simulink model "eVTOL"  (R2025a)
settings: Solver=VariableStepAuto  StartTime=0.0  StopTime=10  RelTol=1e-3
values from neighbouring files (symbols this model uses):
  A = [0 1 0 0 0 0 ... (first row only)    [QRCalculation.m]    (also in QRCalculation2.m = sys.A)
  B = [0 0 0 ... (first row only)    [QRCalculation.m]    (also in QRCalculation2.m = sys.B)
  K = lqr(A,B,Q,R)    [QRCalculation.m]    (also in QRCalculation2.m)
  T = [1 0 0 0 0 0 ... (first row only)    [QRCalculation2.m]
  u0 = [w_trim_vec(1);w_trim_vec(2);w_trim_vec(3);w_trim_vec(4);        eta_trim;eta_trim;eta_trim;eta_trim;        gamma_trim;gamma_trim;gamma_trim;gamma_trim]    [QRCalculation2.m]
undefined symbols (not defined in the file or in its folder): magnitude, Rotor
libraries: aerolibconvert2 x6, shared6dof x1, sharedtransform x1
settings Model: Creator=Administrator  LastModifiedBy=zozo
settings SolverCC: AlgebraicLoopSolver=TrustRegion
settings DataIOCC: ReturnWorkspaceOutputs=off
settings DebuggingCC: UnconnectedInputMsg=warning  UnconnectedOutputMsg=warning  UnconnectedLineMsg=warning  ArithmeticOperatorsInVariantConditions=warning
settings ModelReferenceCC: EnableRefExpFcnMdlSchedulingChecks=on
settings SFSimCC: SimUseLocalCustomCode=off  CustomCodeUndefinedFunction=UseInterfaceOnly
settings RTWCC: RTWUseLocalCustomCode=off  GPUComputeCapability=3.5
settings CodeAppCC: StateflowObjectComments=on

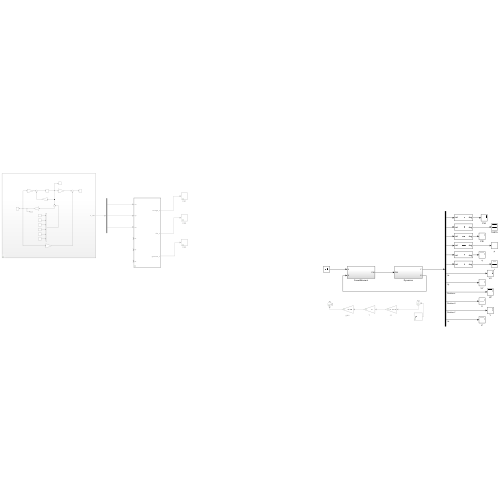
[thumbnail: Simulink's stored preview of the top-level diagram]
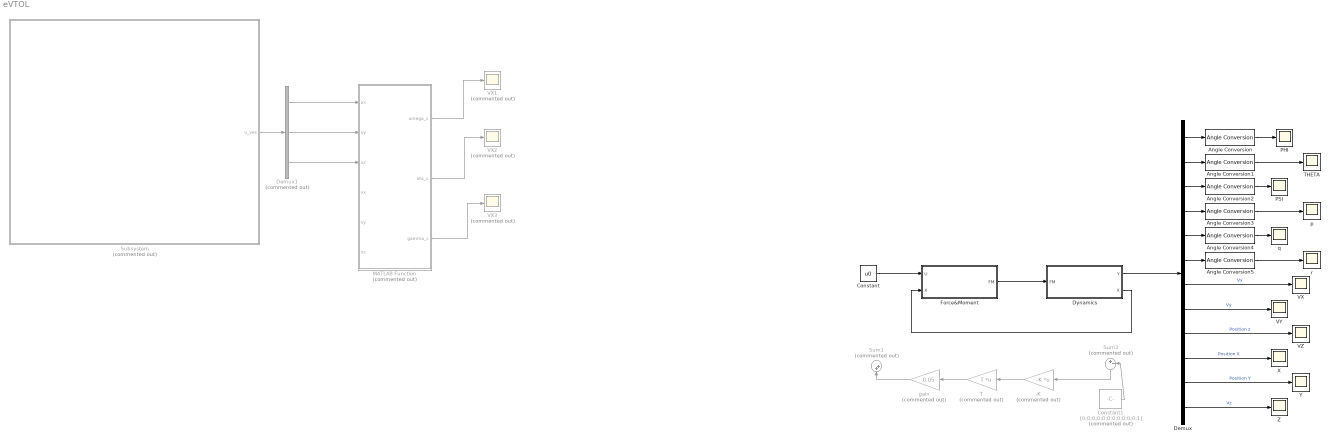
== system eVTOL ==
  -K : Gain  Commented=on  Gain=-K  Multiplication=Matrix(K*u) (u vector)
  Angle Conversion{,1..5} (6 alike) : aerolibconvert2/Angle Conversion  IU=rad  OU=deg
  Constant : Constant  Value=u0
  Constant1 : Constant  Commented=on  Value=[0;0;0;0;0;0;0;0;0;0;0;1]
  Demux : Demux  Outputs=12
  Demux1 : Demux  Commented=on  Outputs=3
  Dynamics : Subsystem
  Force&Moment : Subsystem
  MATLAB Function : MATLAB Function  Commented=on  TreatAsAtomicUnit=on
  PHI : Scope
      settings: ActiveDisplayYMinimum=-1  ActiveDisplayYMaximum=1  DataLoggingVariableName=ScopeData2  DataLoggingSaveFormat=Array
  PSI : Scope
      settings: ActiveDisplayYMinimum=-1  ActiveDisplayYMaximum=1  DataLoggingVariableName=ScopeData3  DataLoggingSaveFormat=Array
  Subsystem : Subsystem  Commented=on
  Sum1 : Sum  Commented=on  Inputs=|++
  Sum3 : Sum  Commented=on  Inputs=|+-
  T : Gain  Commented=on  Gain=T  Multiplication=Matrix(K*u) (u vector)
  THETA : Scope
      settings: ActiveDisplayYMinimum=-1  ActiveDisplayYMaximum=1  DataLoggingVariableName=ScopeData6  DataLoggingSaveFormat=Array
  VX : Scope
      settings: ActiveDisplayYMinimum=-27.584185199806278  ActiveDisplayYMaximum=116.08981655494141  DataLoggingVariableName=ScopeData7  DataLoggingSaveFormat=Array
  VX1 : Scope  Commented=on
      settings: ActiveDisplayYMinimum=7.7412918952680911  ActiveDisplayYMaximum=1205.9707784250681  DataLoggingVariableName=ScopeData15  DataLoggingSaveFormat=Array
  VX2 : Scope  Commented=on
      settings: ActiveDisplayYMinimum=-1.9359903947973216  ActiveDisplayYMaximum=1.846593299645735  DataLoggingVariableName=ScopeData16  DataLoggingSaveFormat=Array
  VX3 : Scope  Commented=on
      settings: ActiveDisplayYMinimum=-3.5342917352885168  ActiveDisplayYMaximum=0.39269908169872469  DataLoggingVariableName=ScopeData17  DataLoggingSaveFormat=Array
  VY : Scope
      settings: ActiveDisplayYMinimum=-36.534383328447007  ActiveDisplayYMaximum=113.30529089895154  DataLoggingVariableName=ScopeData8  DataLoggingSaveFormat=Array
  VZ : Scope
      settings: ActiveDisplayYMinimum=-29.171649220863774  ActiveDisplayYMaximum=3.2412943578737519  DataLoggingVariableName=ScopeData9  DataLoggingSaveFormat=Array
  X : Scope
      settings: ActiveDisplayYMinimum=-75.486762665490659  ActiveDisplayYMaximum=103.49915493683523  DataLoggingVariableName=ScopeData18  DataLoggingSaveFormat=Array
  Y : Scope
      settings: ActiveDisplayYMinimum=-6.2829995724760961  ActiveDisplayYMaximum=56.546996152284883  DataLoggingVariableName=ScopeData11  DataLoggingSaveFormat=Array
  Z : Scope
      settings: ActiveDisplayYMinimum=-90.63503573219765  ActiveDisplayYMaximum=10.070559525799737  DataLoggingSaveFormat=Array
  gain : Gain  Commented=on  Gain=0.05
  p : Scope
      settings: ActiveDisplayYMinimum=-5.4606778718971016E-14  ActiveDisplayYMaximum=1.7107657170555253E-13  DataLoggingSaveFormat=Array
  q : Scope
      settings: ActiveDisplayYMinimum=-7.1821528174857374E-14  ActiveDisplayYMaximum=1.3113311296989755E-14  DataLoggingVariableName=ScopeData4  DataLoggingSaveFormat=Array
  r : Scope
      settings: ActiveDisplayYMinimum=-4.3578208250948042E-29  ActiveDisplayYMaximum=2.2991960417495353E-30  DataLoggingVariableName=ScopeData5  DataLoggingSaveFormat=Array
  wires:
  Force&Moment/1(FM) -> Dynamics/1(FM)
  Dynamics/2(X) -> Force&Moment/2(X)
  Angle Conversion3/1 -> p/1
  Demux/3 -> Angle Conversion2/1
  Demux/2 -> Angle Conversion1/1
  Demux/5 -> Angle Conversion4/1
  Angle Conversion/1 -> PHI/1
  Angle Conversion2/1 -> PSI/1
  Demux/4 -> Angle Conversion3/1
  Angle Conversion4/1 -> q/1
  Angle Conversion5/1 -> r/1
  Demux/6 -> Angle Conversion5/1
  Angle Conversion1/1 -> THETA/1
  Demux/1 -> Angle Conversion/1
  Demux/8 -> VY/1  "Vy"
  Demux/11 -> Y/1  "Position Y"
  Demux1/1 -> MATLAB Function/1(ux)
  Demux1/2 -> MATLAB Function/2(uy)
  Demux1/3 -> MATLAB Function/3(uz)
  Subsystem/1(u_vec) -> Demux1/1
  MATLAB Function/1(omega_c) -> VX1/1
  MATLAB Function/2(eta_c) -> VX2/1
  MATLAB Function/3(gamma_c) -> VX3/1
  Sum3/1 -> -K/1
  -K/1 -> T/1
  Constant1/1 -> Sum3/2
  T/1 -> gain/1
  gain/1 -> Sum1/1
  Demux/9 -> VZ/1  "Position z"
  Demux/12 -> Z/1  "Vz"
  Demux/10 -> X/1  "Position X"
  Demux/7 -> VX/1  "Vx"
  Constant/1 -> Force&Moment/1(U)
  Dynamics/1(Y) -> Demux/1

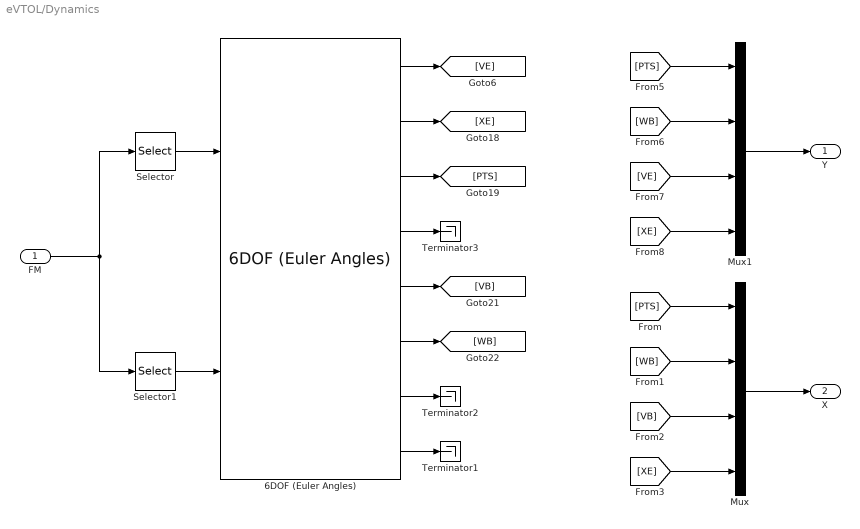
== system eVTOL/Dynamics ==
  FM : Inport
  6DOF (Euler Angles) : shared6dof/6DOF (Euler Angles)  units=Metric (MKS)  mtype=Fixed  rep=Euler Angles  xme_0=Rotor.XE0  Vm_0=Rotor.VB0  eul_0=Rotor.PTS0  pm_0=Rotor.WB0  mass_0=Rotor.MASS  mass_e=0.5  mass_f=2.0  inertia=Rotor.IB  inertia_e=eye(3)  inertia_f=2*eye(3)  k_quat=1.0  vre_flag=on  abi_flag=off  aMode=aMode  xme_statename=''  Vm_statename=''  eul_statename=''  quat_statename=''  pm_statename=''  mass_statename=''
  Mux : Mux
  Mux1 : Mux
  Selector : Selector  InputPortWidth=6  IndexOptions=Index vector (dialog)  Indices=[1:3]  OutputSizes=1
  Selector1 : Selector  InputPortWidth=6  IndexOptions=Index vector (dialog)  Indices=[4:6]  OutputSizes=1
  Terminator1 : Terminator
  Terminator2 : Terminator
  Terminator3 : Terminator
  Y : Outport  VectorParamsAs1DForOutWhenUnconnected=off
  X : Outport  Port=2  VectorParamsAs1DForOutWhenUnconnected=off
  wires:
  6DOF (Euler Angles)/2 -> [XE]
  6DOF (Euler Angles)/3 -> [PTS]
  6DOF (Euler Angles)/4 -> Terminator3/1
  6DOF (Euler Angles)/5 -> [VB]
  6DOF (Euler Angles)/6 -> [WB]
  6DOF (Euler Angles)/1 -> [VE]
  6DOF (Euler Angles)/7 -> Terminator2/1
  6DOF (Euler Angles)/8 -> Terminator1/1
  [XE] -> Mux/4
  [WB] -> Mux/2
  [VB] -> Mux/3
  [PTS] -> Mux/1
  Mux/1 -> X/1
  Selector/1 -> 6DOF (Euler Angles)/1
  FM/1 -> Selector/1, Selector1/1
  Selector1/1 -> 6DOF (Euler Angles)/2
  [XE] -> Mux1/4
  [WB] -> Mux1/2
  [VE] -> Mux1/3
  [PTS] -> Mux1/1
  Mux1/1 -> Y/1

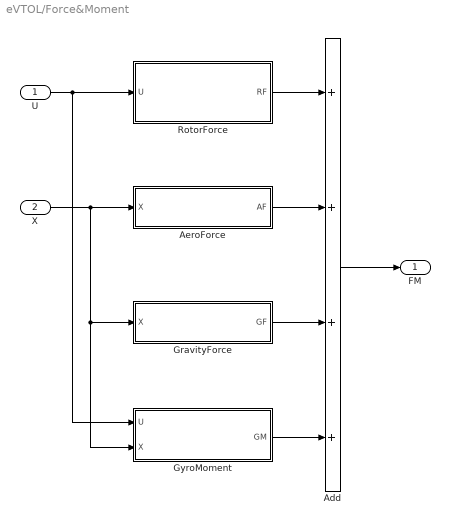
== system eVTOL/Force&Moment ==
  U : Inport
  X : Inport  Port=2
  Add : Sum  Inputs=++++
  AeroForce : Subsystem
  GravityForce : Subsystem
  GyroMoment : Subsystem
  RotorForce : Subsystem
  FM : Outport  VectorParamsAs1DForOutWhenUnconnected=off
  wires:
  Add/1 -> FM/1
  RotorForce/1(RF) -> Add/1
  AeroForce/1(AF) -> Add/2
  U/1 -> GyroMoment/1(U), RotorForce/1(U)
  X/1 -> GyroMoment/2(X), GravityForce/1(X), AeroForce/1(X)
  GravityForce/1(GF) -> Add/3
  GyroMoment/1(GM) -> Add/4

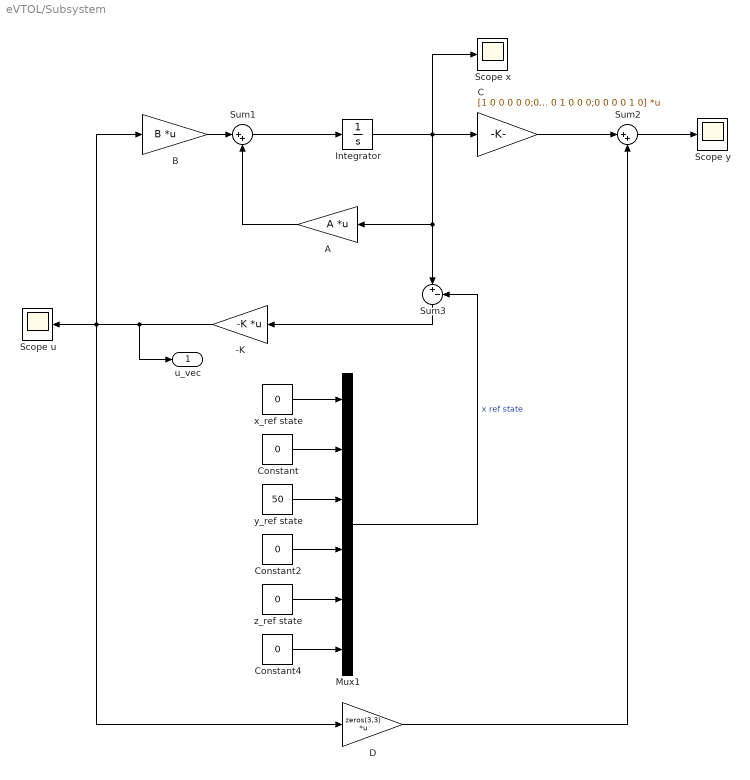
== system eVTOL/Subsystem ==
  -K : Gain  Gain=-K  Multiplication=Matrix(K*u) (u vector)
  A : Gain  Gain=A  Multiplication=Matrix(K*u) (u vector)
  B : Gain  Gain=B  Multiplication=Matrix(K*u) (u vector)
  C : Gain  Gain=[1 0 0 0 0 0;0 0 1 0 0 0;0 0 0 0 1 0]  Multiplication=Matrix(K*u) (u vector)
  Constant : Constant  Value=0
  Constant2 : Constant  Value=0
  Constant4 : Constant  Value=0
  D : Gain  Gain=zeros(3,3)  Multiplication=Matrix(K*u) (u vector)
  Integrator : Integrator  InitialCondition=[0;0;0;0;0;0]
  Mux1 : Mux  Inputs=6
  Scope u : Scope
      settings: ActiveDisplayYMinimum=-225.18678555845298  ActiveDisplayYMaximum=810.69495526932565  DataLoggingVariableName=ScopeData12
  Scope x : Scope
      settings: ActiveDisplayYMinimum=-15.771141244969813  ActiveDisplayYMaximum=129.56230471259059  DataLoggingVariableName=ScopeData13
  Scope y : Scope
      settings: ActiveDisplayYMinimum=-37.880592608204367  ActiveDisplayYMaximum=340.92533347383937  DataLoggingVariableName=ScopeData14
  Sum1 : Sum  Inputs=|++
  Sum2 : Sum  Inputs=|++
  Sum3 : Sum  Inputs=|+-
  x_ref state : Constant  Value=0
  y_ref state : Constant  Value=50
  z_ref state : Constant  Value=0
  u_vec : Outport
  wires:
  B/1 -> Sum1/1
  y_ref state/1 -> Mux1/3
  Sum1/1 -> Integrator/1
  -K/1 -> u_vec/1, B/1, Scope u/1, D/1
  Sum2/1 -> Scope y/1
  x_ref state/1 -> Mux1/1
  Integrator/1 -> Scope x/1, C/1, A/1, Sum3/1
  Constant4/1 -> Mux1/6
  z_ref state/1 -> Mux1/5
  Constant2/1 -> Mux1/4
  A/1 -> Sum1/2
  Sum3/1 -> -K/1
  Constant/1 -> Mux1/2
  D/1 -> Sum2/2
  Mux1/1 -> Sum3/2  "x ref state"
  C/1 -> Sum2/1

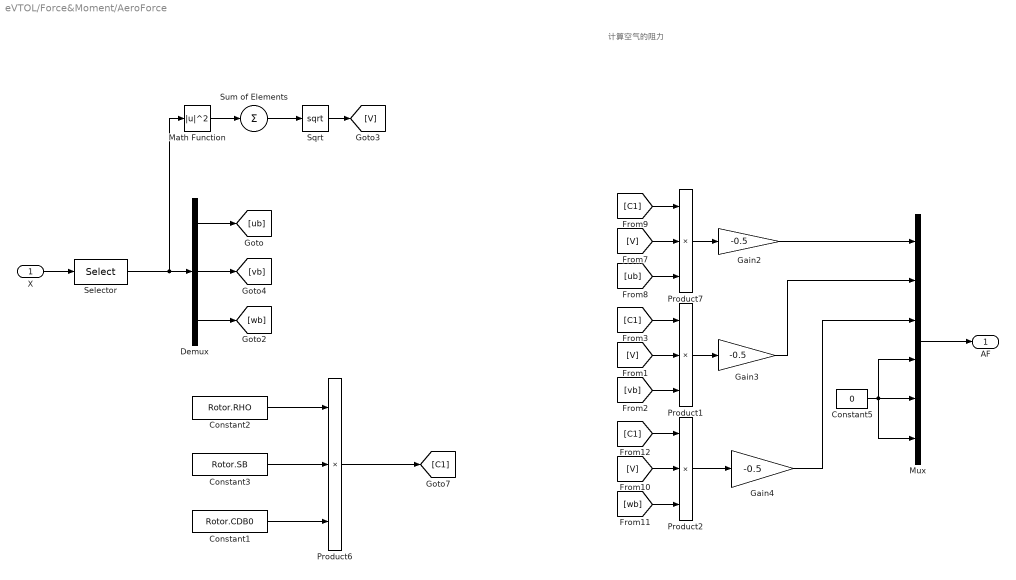
== system eVTOL/Force&Moment/AeroForce ==
  note: 计算空气的阻力
  X : Inport
  Constant1 : Constant  Value=Rotor.CDB0
  Constant2 : Constant  Value=Rotor.RHO
  Constant3 : Constant  Value=Rotor.SB
  Constant5 : Constant  Value=0
  Demux : Demux  Outputs=3
  Gain2 : Gain  Gain=-0.5
  Gain3 : Gain  Gain=-0.5
  Gain4 : Gain  Gain=-0.5
  Math Function : Math  Operator=magnitude^2  SignedPower=on
  Mux : Mux  Inputs=6
  Product{1..2,6..7} (4 alike) : Product  Inputs=3
  Selector : Selector  InputPortWidth=12  IndexOptions=Index vector (dialog)  Indices=[7:9]  OutputSizes=1
  Sqrt : Sqrt
  Sum of Elements : Sum  Inputs=+
  AF : Outport  VectorParamsAs1DForOutWhenUnconnected=off
  wires:
  Mux/1 -> AF/1
  Constant5/1 -> Mux/6, Mux/5, Mux/4
  Demux/3 -> [wb]
  Demux/2 -> [vb]
  Demux/1 -> [ub]
  Math Function/1 -> Sum of Elements/1
  Sqrt/1 -> [V]
  Selector/1 -> Math Function/1, Demux/1
  Gain2/1 -> Mux/1
  X/1 -> Selector/1
  [V] -> Product7/2
  [ub] -> Product7/3
  [C1] -> Product7/1
  Product7/1 -> Gain2/1
  Gain3/1 -> Mux/2
  [V] -> Product1/2
  [vb] -> Product1/3
  [C1] -> Product1/1
  Product1/1 -> Gain3/1
  Gain4/1 -> Mux/3
  [V] -> Product2/2
  [wb] -> Product2/3
  [C1] -> Product2/1
  Product2/1 -> Gain4/1
  Product6/1 -> [C1]
  Constant1/1 -> Product6/3
  Constant2/1 -> Product6/1
  Constant3/1 -> Product6/2
  Sum of Elements/1 -> Sqrt/1

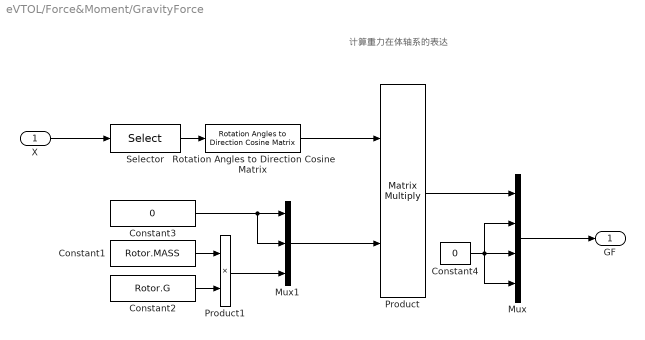
== system eVTOL/Force&Moment/GravityForce ==
  note: 计算重力在体轴系的表达
  X : Inport
  Constant1 : Constant  Value=Rotor.MASS
  Constant2 : Constant  Value=Rotor.G
  Constant3 : Constant  Value=0
  Constant4 : Constant  Value=0
  Mux : Mux
  Mux1 : Mux  Inputs=3
  Product : Product  Inputs=**  Multiplication=Matrix(*)
  Product1 : Product
  Rotation Angles to Direction Cosine Matrix : sharedtransform/Rotation Angles to Direction Cosine Matrix  rotationOrder=ZYX  aMode=aMode
  Selector : Selector  InputPortWidth=12  IndexOptions=Index vector (dialog)  Indices=[3 2 1]  OutputSizes=1
  GF : Outport  VectorParamsAs1DForOutWhenUnconnected=off
  wires:
  Constant3/1 -> Mux1/2, Mux1/1
  Constant1/1 -> Product1/1
  Product/1 -> Mux/1
  Mux1/1 -> Product/2
  Constant2/1 -> Product1/2
  Mux/1 -> GF/1
  Constant4/1 -> Mux/2, Mux/4, Mux/3
  Product1/1 -> Mux1/3
  X/1 -> Selector/1
  Selector/1 -> Rotation Angles to Direction Cosine Matrix/1
  Rotation Angles to Direction Cosine Matrix/1 -> Product/1

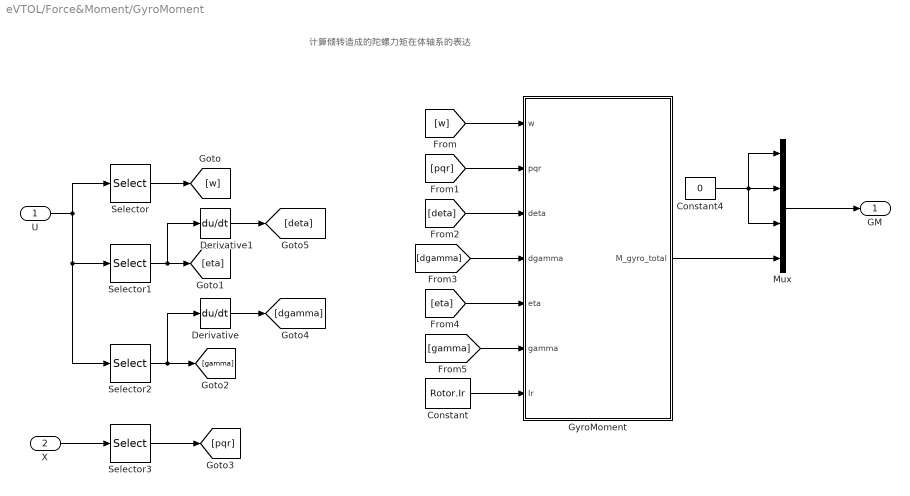
== system eVTOL/Force&Moment/GyroMoment ==
  note: 计算倾转造成的陀螺力矩在体轴系的表达
  U : Inport
  X : Inport  Port=2
  Constant : Constant  Value=Rotor.Ir
  Constant4 : Constant  Value=0
  Derivative : Derivative
  Derivative1 : Derivative
  GyroMoment : MATLAB Function  TreatAsAtomicUnit=on
  Mux : Mux
  Selector : Selector  InputPortWidth=12  IndexOptions=Index vector (dialog)  Indices=[1:4]  OutputSizes=1
  Selector1 : Selector  InputPortWidth=12  IndexOptions=Index vector (dialog)  Indices=[5:8]  OutputSizes=1
  Selector2 : Selector  InputPortWidth=12  IndexOptions=Index vector (dialog)  Indices=[9:12]  OutputSizes=1
  Selector3 : Selector  InputPortWidth=12  IndexOptions=Index vector (dialog)  Indices=[7:9]  OutputSizes=1
  GM : Outport
  wires:
  U/1 -> Selector2/1, Selector1/1, Selector/1
  Selector/1 -> [w]
  Selector1/1 -> Derivative1/1, [eta]
  Selector2/1 -> Derivative/1, [gamma]
  X/1 -> Selector3/1
  Selector3/1 -> [pqr]
  Derivative/1 -> [dgamma]
  Derivative1/1 -> [deta]
  [w] -> GyroMoment/1(w)
  [pqr] -> GyroMoment/2(pqr)
  [deta] -> GyroMoment/3(deta)
  [dgamma] -> GyroMoment/4(dgamma)
  [eta] -> GyroMoment/5(eta)
  [gamma] -> GyroMoment/6(gamma)
  Mux/1 -> GM/1
  GyroMoment/1(M_gyro_total) -> Mux/4
  Constant4/1 -> Mux/3, Mux/2, Mux/1
  Constant/1 -> GyroMoment/7(Ir)

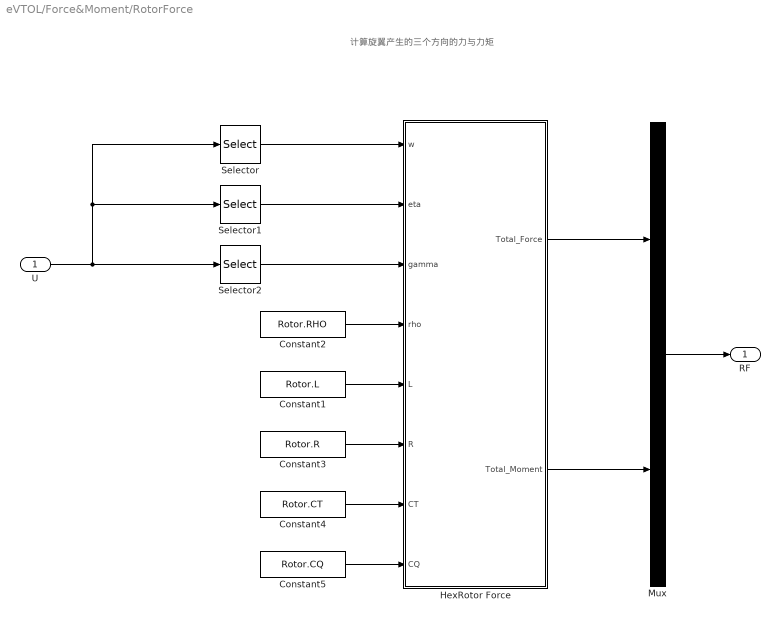
== system eVTOL/Force&Moment/RotorForce ==
  note: 计算旋翼产生的三个方向的力与力矩
  U : Inport
  Constant1 : Constant  Value=Rotor.L
  Constant2 : Constant  Value=Rotor.RHO
  Constant3 : Constant  Value=Rotor.R
  Constant4 : Constant  Value=Rotor.CT
  Constant5 : Constant  Value=Rotor.CQ
  HexRotor Force : MATLAB Function  TreatAsAtomicUnit=on
  Mux : Mux  Inputs=2
  Selector : Selector  InputPortWidth=12  IndexOptions=Index vector (dialog)  Indices=[1:4]  OutputSizes=1
  Selector1 : Selector  InputPortWidth=12  IndexOptions=Index vector (dialog)  Indices=[5:8]  OutputSizes=1
  Selector2 : Selector  InputPortWidth=12  IndexOptions=Index vector (dialog)  Indices=[9:12]  OutputSizes=1
  RF : Outport  VectorParamsAs1DForOutWhenUnconnected=off
  wires:
  Mux/1 -> RF/1
  Selector/1 -> HexRotor Force/1(w)
  HexRotor Force/1(Total_Force) -> Mux/1
  HexRotor Force/2(Total_Moment) -> Mux/2
  U/1 -> Selector2/1, Selector1/1, Selector/1
  Constant2/1 -> HexRotor Force/4(rho)
  Constant1/1 -> HexRotor Force/5(L)
  Constant3/1 -> HexRotor Force/6(R)
  Constant4/1 -> HexRotor Force/7(CT)
  Constant5/1 -> HexRotor Force/8(CQ)
  Selector1/1 -> HexRotor Force/2(eta)
  Selector2/1 -> HexRotor Force/3(gamma)

== matlab function eVTOL/MATLAB Function ==
  data: ux input; omega_c output; uy input; uz input; eta_c output; gamma_c output; vx input; vy input; vz input
function [omega_c, eta_c, gamma_c] = allocator(ux, uy, uz, vx, vy, vz)
%#codegen

rho = 1.225;
g   = 9.81;
m   = 190.4057;
CT  = 0.012;
R   = 0.9;
A   = pi*R^2;

u_x = ux+0.146*vx;
u_y = uy+0.074*vy;
u_z = uz-0*vz;

% total thrust
Td = m * sqrt(u_x^2 + u_y^2 + (u_z + g)^2);

% rotor speed
omega_c = sqrt(Td / (4*rho*A*R^2*CT));

% common tilt angles
eta_c   = -atan2(u_x, u_z + g);
gamma_c = atan2(u_y, u_z + g);

== matlab function eVTOL/Force&Moment/GyroMoment/GyroMoment ==
  data: w input; M_gyro_total output; pqr input; deta input; dgamma input; eta input; gamma input; Ir input
function M_gyro_total = calc_gyro_moment(w, pqr, deta, dgamma, eta, gamma, Ir)
% w: 电机转速 [w1; w2; w3; w4]
% pqr: 机体角速度 [p; q; r]
% deta, dgamma: 机臂和推力关节的角速度 (d(eta)/dt, d(gamma)/dt)
% eta, gamma: 当前的角度

M_gyro_total = [0; 0; 0];
dir = [1; -1; 1; -1]; % 旋翼转向

for i = 1:4
    % 1. 计算坐标变换矩阵 (同之前逻辑)
    R_P2A = [1, 0, 0; 0, cos(gamma(i)), -sin(gamma(i)); 0, sin(gamma(i)), cos(gamma(i))];
    R_A2B = [cos(eta(i)), 0, sin(eta(i)); 0, 1, 0; -sin(eta(i)), 0, cos(eta(i))];
    R_P2B = R_A2B * R_P2A;

    % 2. 计算旋翼在机身坐标系下的角动量方向
    % 旋翼在 Push 系下沿 Z 轴旋转，角速度为 dir(i)*w(i)
    H_p_body = R_P2B * [0; 0; dir(i) * w(i) * Ir];

    % 3. 计算旋翼组件相对于惯性空间的综合角速度 (投影在机身坐标系)
    % 机体转动 + 机臂转动(绕Yb) + 推力关节转动(经过R_A2B变换后的Xa)
    omega_comp_i = pqr + [0; deta(i); 0] + R_A2B * [dgamma(i); 0; 0];

    % 4. 计算该旋翼的陀螺力矩并累加
    % M = omega x H
    M_gyro_total = M_gyro_total + cross(omega_comp_i, H_p_body);
end

== matlab function eVTOL/Force&Moment/RotorForce/HexRotor Force ==
  data: w input; Total_Force output; eta input; gamma input; Total_Moment output; rho input; L input; R input; CT input; CQ input
function [Total_Force, Total_Moment] = RotorForce(w, eta, gamma, rho, L, R, CT, CQ)
% w: 4x1 电机转速向量 [w1; w2; w3; w4]
% eta: 4x1 机臂倾斜角向量
% params: 结构体，包含 L (臂长), CT (推力系数), CQ (阻力系数), rho (空气密度), R (半径), A (面积)

% 初始化总力和力矩
Total_Force = [0; 0; 0];
Total_Moment = [0; 0; 0];


% 旋翼位置分配 (假设 X型布局)
% r_i: 各旋翼相对于重心的位置矢量 

A = pi*R^2;

x = L/sqrt(2);
y = L/sqrt(2);

% 无人机旋翼标号定义
%  4       1
%    -   - 
%      o
%    -   -
%  3       2

r_pos = [ x, -x, -x,  x;  % x 轴位置
          y,  y, -y, -y;  % y 轴位置
          0,  0,  0,  0]; % z 轴位置 (假设在同一平面)

% 旋翼转向系数 (1代表顺时针，-1代表逆时针)
% 注意：阻力矩方向与转向相反
dir = [1; -1; 1; -1]; 

for i = 1:4
    %% 1. 计算单个旋翼在自身坐标系下的受力 
    Ti = rho * A * (w(i) * R)^2 * CT;
    Qi = rho * A * (w(i) * R)^2 * R * CQ;
    
    % 推力矢量 (沿 Zp 轴)
    T_Pi = [0; 0; -Ti]; % Z轴朝下，推力向上则为负 
    % 反扭矩矢量 (沿 Zp 轴)
    Q_Pi = [0; 0; dir(i) * Qi];

    %% 2. 坐标变换矩阵
    % Push to Arm (绕 X 轴)
    R_P2A = [1, 0, 0; 
             0, cos(gamma(i)), -sin(gamma(i)); 
             0, sin(gamma(i)), cos(gamma(i))];
    
    % Arm to Body (绕 Y 轴)
    R_A2B = [cos(eta(i)), 0, sin(eta(i)); 
             0, 1, 0; 
             -sin(eta(i)), 0, cos(eta(i))];
    
    % 复合变换阵
    R_P2B = R_A2B * R_P2A;

    %% 3. 转换到机体坐标系
    F_Bi = R_P2B * T_Pi; % 该旋翼产生的推力在机体系下的分量
    Q_Bi = R_P2B * Q_Pi; % 该旋翼产生的反扭力矩在机体系下的分量
    
    %% 4. 累加总力和总力矩
    Total_Force = Total_Force + F_Bi;
    
    % 总力矩 = sum(力臂 x 推力矢量 + 阻力矩矢量)
    Total_Moment = Total_Moment + cross(r_pos(:,i), F_Bi) + Q_Bi;
end
